simulink model "PassStFtHolderChk"  (R2018b)
settings: Solver=FixedStepDiscrete  StartTime=0.0  StopTime=10.0  FixedStep=0.01  RelTol=1e-3
libraries: simulink x1
settings Model: Creator=sn2xws  LastModifiedBy=sn2xws
settings DataIOCC: SaveFormat=StructureWithTime
settings OptimizationCC: DefaultParameterBehavior=Inlined  EnhancedBackFolding=on  PassReuseOutputArgsAs=Individual arguments  ZeroExternalMemoryAtStartup=off  ZeroInternalMemoryAtStartup=off  OptimizeBlockOrder=speed  DifferentSizesBufferReuse=on  OptimizationCustomize=off
settings DebuggingCC: ParameterTunabilityLossMsg=error
settings ModelReferenceCC: ModelReferenceNumInstancesAllowed=Single
settings SFSimCC: MATLABDynamicMemAlloc=off
settings RTWCC: SystemTargetFile=autosar.tlc  GenCodeOnly=on  TemplateMakefile=ert_default_tmf  Description=AUTOSAR  GenerateReport=on  IncludeHyperlinkInReport=on  LaunchReport=on  GenerateTraceInfo=on  GenerateTraceReport=on  GenerateTraceReportSl=on  GenerateTraceReportSf=on  GenerateTraceReportEml=on
settings CodeAppCC: ForceParamTrailComments=on  IgnoreCustomStorageClasses=off  OperatorAnnotations=on  SimulinkDataObjDesc=on  SFDataObjDesc=on  InsertBlockDesc=on
settings STFCustomTargetCC: TargetLangStandard=C99 (ISO)  MultiwordLength=256  ParMdlRefBuildCompliant=on  CompOptLevelCompliant=on  IncludeMdlTerminateFcn=off  CombineOutputUpdateFcns=on  SuppressErrorStatus=on  ERTCustomFileBanners=on  SupportNonFinite=off  SupportComplex=off  SupportContinuousTime=off  SupportNonInlinedSFcns=off  RemoveResetFunc=on  MATLABClassNameForMDSCustomization=Simulink.SoftwareTarget.ERTCustomization  AutosarCompliant=on  UseToolchainInfoCompliant=on  LookupTableObjectStructAxisOrder=2,1,3,4,...  LUTObjectStructOrderEvenSpacing=Size,Table,Breakpoints  SystemTargetFile=autosar.tlc
settings ERTTargetCC: TargetLangStandard=C99 (ISO)  ConcurrentExecutionCompliant=off  IncludeMdlTerminateFcn=off  SuppressErrorStatus=on  SupportNonFinite=off  SupportComplex=off  ModelStepFunctionPrototypeControlCompliant=off  CPPClassGenCompliant=off  AutosarCompliant=on  LookupTableObjectStructAxisOrder=2,1,3,4,...  LUTObjectStructOrderEvenSpacing=Size,Table,Breakpoints  InlinedParameterPlacement=NonHierarchical  ERTCustomFileTemplate=example_file_process.tlc  ERTFilePackagingFormat=Compact

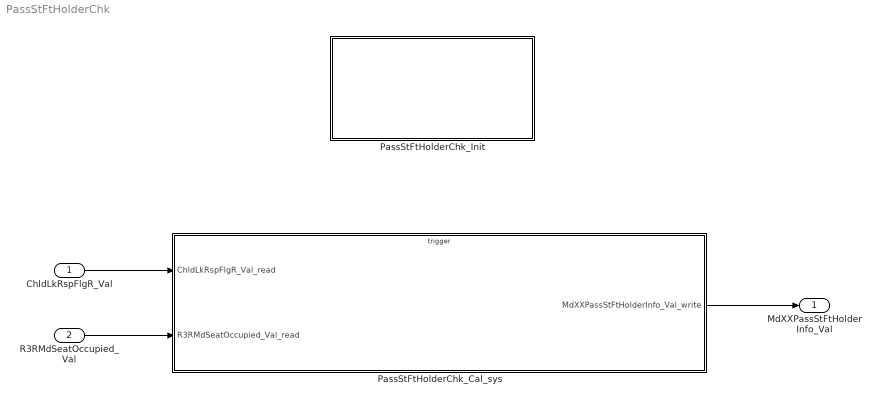
== system PassStFtHolderChk ==
  ChldLkRspFlgR_Val : Inport  OutDataTypeStr=boolean  PortDimensions=1
  R3RMdSeatOccupied_Val : Inport  Port=2  OutDataTypeStr=boolean  PortDimensions=1
  PassStFtHolderChk_Cal_sys : Subsystem
  PassStFtHolderChk_Init : Subsystem
  MdXXPassStFtHolderInfo_Val : Outport  OutDataTypeStr=uint32  PortDimensions=1
  wires:
  PassStFtHolderChk_Cal_sys/1(MdXXPassStFtHolderInfo_Val_write) -> MdXXPassStFtHolderInfo_Val/1
  ChldLkRspFlgR_Val/1 -> PassStFtHolderChk_Cal_sys/1(ChldLkRspFlgR_Val_read)
  R3RMdSeatOccupied_Val/1 -> PassStFtHolderChk_Cal_sys/2(R3RMdSeatOccupied_Val_read)

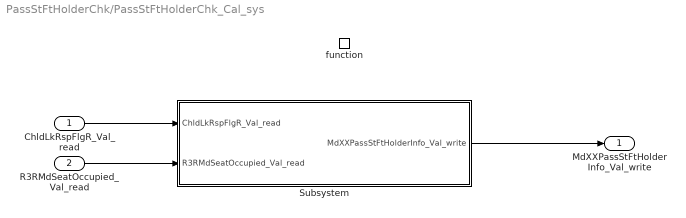
== system PassStFtHolderChk/PassStFtHolderChk_Cal_sys ==
  ChldLkRspFlgR_Val_read : Inport
  R3RMdSeatOccupied_Val_read : Inport  Port=2
  function : TriggerPort  TriggerType=function-call  IsSimulinkFunction=on  FunctionName=PassStFtHolderChk_Cal  VariantControl=(inherit)
  Subsystem : Subsystem
  MdXXPassStFtHolderInfo_Val_write : Outport
      settings: EnsureOutportIsVirtual=on
  wires:
  ChldLkRspFlgR_Val_read/1 -> Subsystem/1(ChldLkRspFlgR_Val_read)
  R3RMdSeatOccupied_Val_read/1 -> Subsystem/2(R3RMdSeatOccupied_Val_read)
  Subsystem/1(MdXXPassStFtHolderInfo_Val_write) -> MdXXPassStFtHolderInfo_Val_write/1

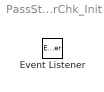
== system PassStFtHolderChk/PassStFtHolderChk_Init ==
  Event Listener : EventListener  EventName=reset

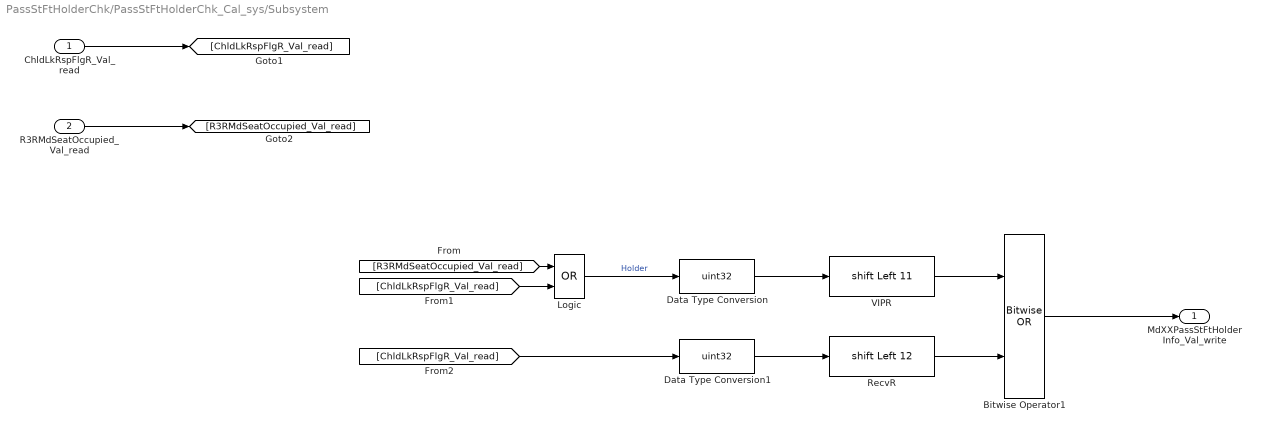
== system PassStFtHolderChk/PassStFtHolderChk_Cal_sys/Subsystem ==
  ChldLkRspFlgR_Val_read : Inport
  R3RMdSeatOccupied_Val_read : Inport  Port=2
  Bitwise Operator1 : simulink/Logic and Bit Operations/Bitwise Operator  logicop=OR  UseBitMask=off  NumInputPorts=2  BitMask=bin2dec('11011001')  BitMaskRealWorld=Stored Integer
  Data Type Conversion : DataTypeConversion  OutDataTypeStr=uint32
  Data Type Conversion1 : DataTypeConversion  OutDataTypeStr=uint32
  Logic : Logic  Operator=OR  AllPortsSameDT=off  OutDataTypeStr=boolean
  RecvR : ArithShift  BitShiftNumber=12  BitShiftDirection=Left
  VIPR : ArithShift  BitShiftNumber=11  BitShiftDirection=Left
  MdXXPassStFtHolderInfo_Val_write : Outport
      settings: EnsureOutportIsVirtual=on
  wires:
  Data Type Conversion1/1 -> RecvR/1
  RecvR/1 -> Bitwise Operator1/2
  Bitwise Operator1/1 -> MdXXPassStFtHolderInfo_Val_write/1
  Data Type Conversion/1 -> VIPR/1
  [ChldLkRspFlgR_Val_read] -> Logic/2
  VIPR/1 -> Bitwise Operator1/1
  [ChldLkRspFlgR_Val_read] -> Data Type Conversion1/1
  [R3RMdSeatOccupied_Val_read] -> Logic/1
  Logic/1 -> Data Type Conversion/1  "Holder"
  ChldLkRspFlgR_Val_read/1 -> [ChldLkRspFlgR_Val_read]
  R3RMdSeatOccupied_Val_read/1 -> [R3RMdSeatOccupied_Val_read]
